simulink subsystem "ControlBA"  (R2023b)
settings: Solver=VariableStepAuto  StartTime=0.0  StopTime=10.0  RelTol=1e-3
settings Model: Creator=Felix  LastModifiedBy=Felix

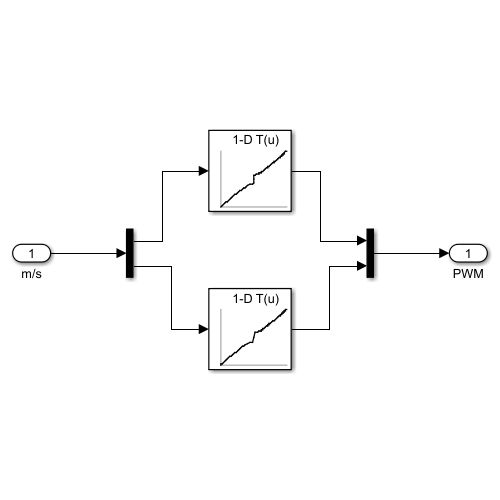
[thumbnail: Simulink's stored preview of the top-level diagram]
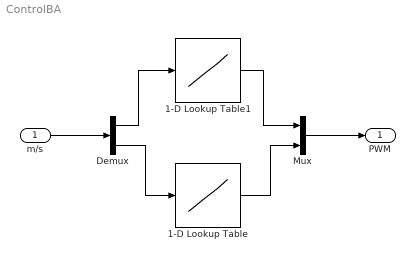
== system ControlBA ==
  m/s : Inport
  1-D Lookup Table : Lookup_n-D  NumberOfTableDimensions=1  BreakpointsForDimension1=[-0.48464298248291;-0.473752021789551;-0.460138320922852;-0.446524620056152;-0.43018913269043;-0.413852691650391;-0.39887809753418;-0.382539749145508;-0.364845275878906;-0.349868774414063;-0.332170486450195;-0.313112258911133;-0.295413970947266;-0.279077529907227;-0.260019302368164;-0.242321014404297;-0.225986480712891;-0.206924438476563;-0.190593719482422;-0.172889709472656;-0.153833389282227;-0.136137008666992;-0.115715026855469;-0.0898494720458984;-0.0449256896972656;-0.00272178649902344;0;0.0190589968115091;0.0612610578536987;0.0884881988167763;0.103463113307953;0.11707666516304;0.129328966140747;0.140219688415527;0.149749279022217;0.160640060901642;0.171531021595001;0.181060433387756;0.191951274871826;0.202842235565186;0.213732957839966;0.223262548446655;0.236876010894775;0.243682861328125;0.254573822021484;0.268187284469605;0.277716875076294;0.289968967437744;0.299498558044434;0.309028148651123;0.324002742767334;0.332170963287354;0.343061923980713;0.352591514587402;0.362120628356934;0.373012065887451;0.382541179656982;0.3934326171875;0.401599884033203;0.412490844726563;0.423381805419922;0.434272766113281;0.441080093383789;0.451971054077148;0.460138320922852;0.471029281616211;0.477836608886719;0.483281135559082;0.491450309753418;0.496894836425781]  Table=[-254;-245.52;-237.03;-228.55;-220.07;-211.58;-203.1;-194.62;-186.13;-177.65;-169.17;-160.68;-152.2;-143.72;-135.23;-126.75;-118.27;-109.78;-101.3;-92.82;-84.33;-75.85;-67.37;-58.88;-50.4;-41.92;0;40.8000068664551;45.9000015258789;50.9999961853027;56.1000061035156;61.2000007629395;66.2999954223633;71.4000091552734;76.5;81.6000137329102;86.7000122070313;91.8000030517578;96.9000015258789;101.999992370605;107.099990844727;112.200012207031;117.300010681152;122.400001525879;127.5;132.599990844727;137.70002746582;142.800018310547;147.900009155273;153;158.100006103516;163.200012207031;168.300003051758;173.400009155273;178.5;183.599990844727;188.700012207031;193.800018310547;198.900009155273;204;209.099990844727;214.200012207031;219.300003051758;224.399993896484;229.5;234.599990844727;239.700012207031;244.800003051758;249.900009155273;255]  InternalRulePriority=Speed  RndMeth=Simplest
  1-D Lookup Table1 : Lookup_n-D  NumberOfTableDimensions=1  BreakpointsForDimension1=[-0.48736572265625;-0.472390174865723;-0.45877742767334;-0.443802833557129;-0.428827285766602;-0.412490844726563;-0.396156311035156;-0.378456115722656;-0.360759735107422;-0.343061447143555;-0.32536506652832;-0.309028625488281;-0.291328430175781;-0.27363395690918;-0.25593376159668;-0.239599227905273;-0.220541000366211;-0.204202651977539;-0.183782577514648;-0.16880989074707;-0.149747848510742;-0.130691528320313;-0.111629486083984;-0.0925731658935547;-0.0585384368896484;-0.0163345336914063;-0.00136184692382813;0;0.0108908545225859;0.0245044250041246;0.0476474836468697;0.0707905516028404;0.087126836180687;0.100740432739258;0.114353954792023;0.125244826078415;0.136135637760162;0.145665228366852;0.157917439937592;0.167446851730347;0.176976442337036;0.186505913734436;0.197396755218506;0.206926107406616;0.217817068099976;0.230069398880005;0.239598751068115;0.247766971588135;0.260019063949585;0.270910024642944;0.280439615249634;0.289969205856323;0.299498558044434;0.313111782073975;0.322641372680664;0.333532810211182;0.341700553894043;0.352591514587402;0.362120628356934;0.371650695800781;0.381179809570313;0.390708923339844;0.40160083770752;0.411129951477051;0.420659065246582;0.431550025939941;0.439718246459961;0.446524620056152;0.456055641174316;0.464221954345703;0.471029281616211;0.480559349060059;0.488726615905762]  Table=[-254;-245.52;-237.03;-228.55;-220.07;-211.58;-203.1;-194.62;-186.13;-177.65;-169.17;-160.68;-152.2;-143.72;-135.23;-126.75;-118.27;-109.78;-101.3;-92.82;-84.33;-75.85;-67.37;-58.88;-50.4;-41.92;-33.43;0;30.6000156402588;35.6999969482422;40.8000068664551;45.9000015258789;50.9999961853027;56.1000061035156;61.2000007629395;66.2999954223633;71.4000091552734;76.5;81.6000137329102;86.7000122070313;91.8000030517578;96.9000015258789;101.999992370605;107.099990844727;112.200012207031;117.300010681152;122.400001525879;127.5;132.599990844727;137.70002746582;142.800018310547;147.900009155273;153;158.100006103516;163.200012207031;168.300003051758;173.400009155273;178.5;183.599990844727;188.700012207031;193.800018310547;198.900009155273;204;209.099990844727;214.200012207031;219.300003051758;224.399993896484;229.5;234.599990844727;239.700012207031;244.800003051758;249.900009155273;255]  InternalRulePriority=Speed  RndMeth=Simplest
  Demux : Demux  Outputs=2
  Mux : Mux  Inputs=2
  PWM : Outport
  wires:
  1-D Lookup Table1/1 -> Mux/1
  1-D Lookup Table/1 -> Mux/2
  Demux/2 -> 1-D Lookup Table/1
  Demux/1 -> 1-D Lookup Table1/1
  Mux/1 -> PWM/1
  m/s/1 -> Demux/1
